simulink model "Loops"  (R2025b)
settings: Solver=FixedStepDiscrete  StartTime=0.0  StopTime=10.0  FixedStep=0.01  RelTol=1e-3
settings Model: Creator=soura  LastModifiedBy=soura

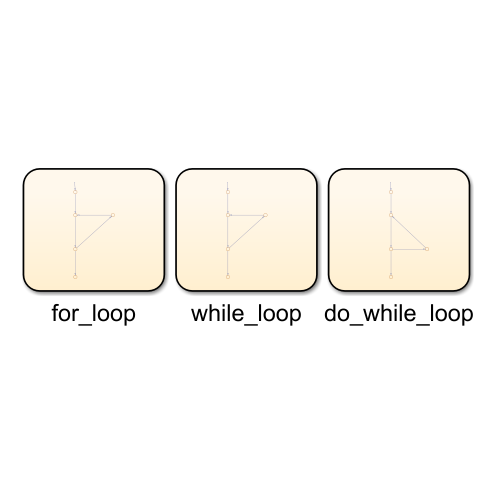
[thumbnail: Simulink's stored preview of the top-level diagram]
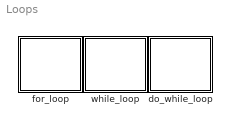
== system Loops ==
  do_while_loop : Stateflow chart  TreatAsAtomicUnit=on
  for_loop : Stateflow chart  TreatAsAtomicUnit=on
  while_loop : Stateflow chart  TreatAsAtomicUnit=on

== stateflow chart Loops/while_loop ==
  (default) -> (junction 4)
  (junction 4) -> (junction 1) : {cond=0;}
  (junction 3) -> (junction 1) : {cond=cond+1;}
  (junction 2) -> (junction 3) [order 1] : [cond<10]
  (junction 1) -> (junction 2)
  (junction 2) -> (junction 9) [order 2]
  data: idx local uint8 size=1

== stateflow chart Loops/do_while_loop ==
  (default) -> (junction 4)
  (junction 4) -> (junction 1) : {cond=0;}
  (junction 3) -> (junction 1)
  (junction 1) -> (junction 2) : {cond=cond+1;}
  (junction 2) -> (junction 3) [order 1] : [cond<10]
  (junction 2) -> (junction 9) [order 2]
  data: idx local uint8 size=1

== stateflow chart Loops/for_loop ==
  (default) -> (junction 4)
  (junction 4) -> (junction 1) : {idx=0;}
  (junction 3) -> (junction 1) : {idx=idx+1;}
  (junction 1) -> (junction 2)
  (junction 2) -> (junction 3) [order 1] : [idx<10]
  (junction 2) -> (junction 9) [order 2]
  data: idx local uint8 size=1
